simulink model "Position_Control_Sim_01"  (R2025b)
settings: Solver=FixedStepAuto  StartTime=0.0  StopTime=inf  FixedStep=time_step  RelTol=1e-3
values from neighbouring files (symbols this model uses):
  I_max_XY = 5    [Position_Control_Main.m]
  I_max_Z = 1    [Position_Control_Main.m]
  MOT_THST_HOVER_MCS = 1470    [Position_Control_Main.m]
  STABILIZE = 1100    [Position_Control_Main.m]
  time_step = 1/80    (= 0.0125)    [Position_Control_Main.m]
undefined symbols (not defined in the file or in its folder): Data, Data_SL_Info, DiscIntNeverNeededParam
libraries: robotlib x5, sharedtransform x1, aerolibanimutils x1
settings Model: Creator=lirangoshen  LastModifiedBy=lirangoshen
settings DataIOCC: LimitDataPoints=on  MaxDataPoints=10000
settings OptimizationCC: EnhancedBackFolding=on  PassReuseOutputArgsAs=Individual arguments  ZeroExternalMemoryAtStartup=off  ZeroInternalMemoryAtStartup=off  MaxStackSize=64  OptimizeBlockOrder=speed  DifferentSizesBufferReuse=on  OptimizationCustomize=off  EfficientTunableParamExpr=on
settings DebuggingCC: ParameterTunabilityLossMsg=error
settings HardwareCC: ProdBitPerPointer=32.0  ProdBitPerSizeT=32.0  ProdBitPerPtrDiffT=32.0  ProdLargestAtomicFloat=None  ProdIntDivRoundTo=Undefined  ProdEndianess=Unspecified  ProdWordSize=32.0  ProdHWDeviceType=Generic->Unspecified (assume 32-bit Generic)
settings SFSimCC: MATLABDynamicMemAlloc=off
settings RTWCC: SystemTargetFile=ert.tlc  HardwareBoard=Robot Operating System (ROS)  TLCOptions="-aInlineSetEventsForThisBaseRateFcn=TLC_FALSE -aSuppressMultiTaskScheduler=TLC_FALSE  -aRateBasedStepFcn=0"  TemplateMakefile=ert_default_tmf  Toolchain=Catkin  TargetLang=C++  GPUComputeCapability=3.5  Description=Embedded Coder
settings CodeAppCC: ForceParamTrailComments=on  IgnoreCustomStorageClasses=off  OperatorAnnotations=on  SimulinkDataObjDesc=on  SFDataObjDesc=on  InsertBlockDesc=on
settings ERTTargetCC: InlinedParameterPlacement=Hierarchical  DynamicArrayContainerType=coder::array

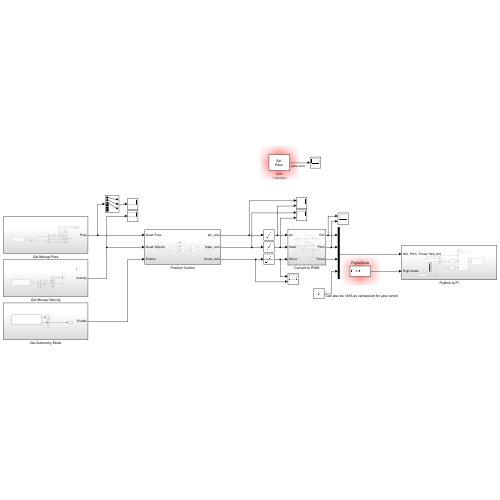
[thumbnail: Simulink's stored preview of the top-level diagram]
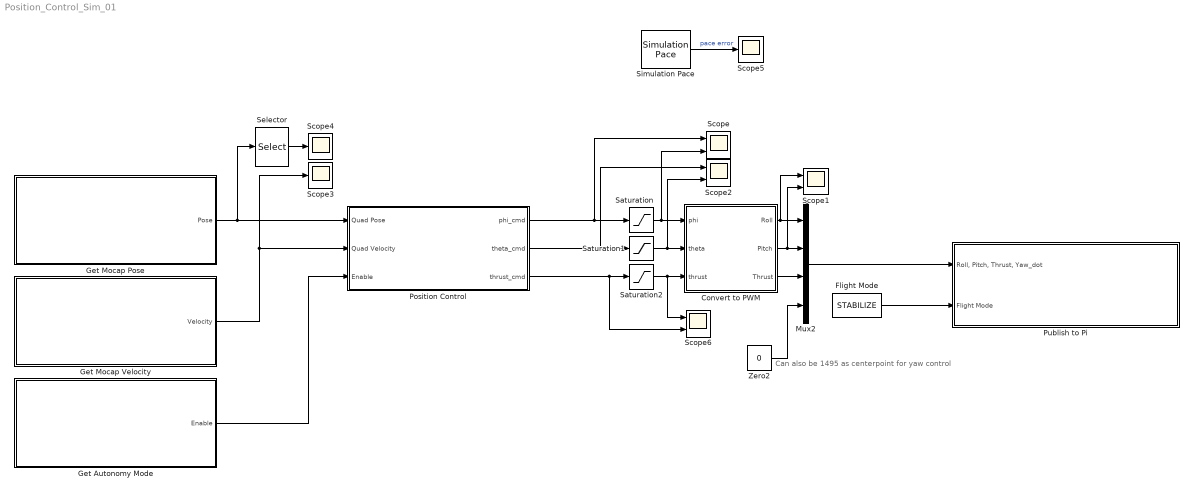
== system Position_Control_Sim_01 ==
  note: Can also be 1495 as centerpoint for yaw control
  Convert to PWM : Subsystem
  Flight Mode : Constant  Value=STABILIZE  OutDataTypeStr=Inherit: Inherit via back propagation
  Get Autonomy Mode : Subsystem
  Get Mocap Pose : Subsystem
  Get Mocap Velocity : Subsystem
  Mux2 : Mux
  Position Control : Subsystem
  Publish to Pi : Subsystem
  Saturation : Saturate  UpperLimit=10  LowerLimit=-10
  Saturation1 : Saturate  UpperLimit=10  LowerLimit=-10
  Saturation2 : Saturate  UpperLimit=3  LowerLimit=-3
  Scope{,1..2,6} (4 alike) : Scope  NumInputPorts=2
      Scope settings: ActiveDisplayYMinimum=-38.87191  ActiveDisplayYMaximum=29.85251
      Scope1 settings: ActiveDisplayYMinimum=1289.66667  ActiveDisplayYMaximum=1706.33333  DataLoggingVariableName=ScopeData2
      Scope2 settings: ActiveDisplayYMinimum=-6.82058  ActiveDisplayYMaximum=8.21599  DataLoggingVariableName=ScopeData3
      Scope6 settings: ActiveDisplayYMinimum=-6.19589  ActiveDisplayYMaximum=6.86106  DataLoggingVariableName=ScopeData7
  Scope3 : Scope
      settings: ActiveDisplayYMinimum=-0.74653  ActiveDisplayYMaximum=0.88268  DataLoggingVariableName=ScopeData4
  Scope4 : Scope
      settings: ActiveDisplayYMinimum=-0.65562  ActiveDisplayYMaximum=1.49202  DataLoggingVariableName=ScopeData5
  Scope5 : Scope
      settings: ActiveDisplayYMinimum=-1  ActiveDisplayYMaximum=1  DataLoggingVariableName=ScopeData6
  Selector : Selector  InputPortWidth=6  IndexOptions=Index vector (dialog)  Indices=1:3  OutputSizes=1
  Simulation Pace : aerolibanimutils/Simulation Pace  SimulationPace=1  SleepMode=Auto  OutputPaceError=on  SampleTime=time_step
  Zero2 : Constant  Value=0  OutDataTypeStr=Inherit: Inherit via back propagation
  wires:
  Flight Mode/1 -> Publish to Pi/2(Flight Mode)
  Position Control/3(thrust_cmd) -> Scope6/2, Saturation2/1
  Convert to PWM/3(Thrust) -> Mux2/3
  Saturation/1 -> Scope/2, Convert to PWM/1(phi)
  Get Mocap Pose/1(Pose) -> Selector/1, Position Control/1(Quad Pose)
  Get Mocap Velocity/1(Velocity) -> Position Control/2(Quad Velocity), Scope3/1
  Convert to PWM/2(Pitch) -> Scope1/2, Mux2/2
  Saturation1/1 -> Scope2/2, Convert to PWM/2(theta)
  Position Control/2(theta_cmd) -> Scope2/1, Saturation1/1
  Saturation2/1 -> Scope6/1, Convert to PWM/3(thrust)
  Zero2/1 -> Mux2/4
  Mux2/1 -> Publish to Pi/1("Roll, Pitch, Thrust, Yaw_dot")
  Selector/1 -> Scope4/1
  Simulation Pace/1 -> Scope5/1  "pace error"
  Get Autonomy Mode/1(Enable) -> Position Control/3(Enable)
  Convert to PWM/1(Roll) -> Mux2/1, Scope1/1
  Position Control/1(phi_cmd) -> Scope/1, Saturation/1

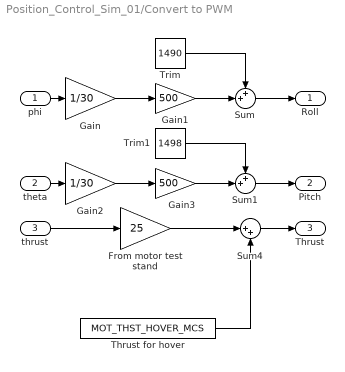
== system Position_Control_Sim_01/Convert to PWM ==
  phi : Inport
  theta : Inport  Port=2
  thrust : Inport  Port=3
  From motor test stand : Gain  Gain=25
  Gain : Gain  Gain=1/30
  Gain1 : Gain  Gain=500
  Gain2 : Gain  Gain=1/30
  Gain3 : Gain  Gain=500
  Sum : Sum  Inputs=++|
  Sum1 : Sum  Inputs=++|
  Sum4 : Sum  Inputs=|++
  Thrust for hover : Constant  Value=MOT_THST_HOVER_MCS
  Trim : Constant  Value=1490
  Trim1 : Constant  Value=1498
  Roll : Outport
  Pitch : Outport  Port=2
  Thrust : Outport  Port=3
  wires:
  phi/1 -> Gain/1
  Gain/1 -> Gain1/1
  Gain1/1 -> Sum/2
  theta/1 -> Gain2/1
  Gain2/1 -> Gain3/1
  Gain3/1 -> Sum1/2
  Sum1/1 -> Pitch/1
  Sum/1 -> Roll/1
  Trim/1 -> Sum/1
  Sum4/1 -> Thrust/1
  Thrust for hover/1 -> Sum4/2
  From motor test stand/1 -> Sum4/1
  Trim1/1 -> Sum1/1
  thrust/1 -> From motor test stand/1

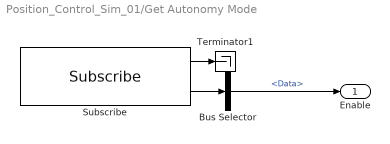
== system Position_Control_Sim_01/Get Autonomy Mode ==
  Bus Selector : BusSelector  OutputSignals=Data
  Subscribe : robotlib/Subscribe  topicSource=Select from ROS network  topic=/autonomy_enable  messageType=std_msgs/Bool  SampleTime=-1  legacyBusStruct=off  messageQueueLength=1
  Terminator1 : Terminator
  Enable : Outport
  wires:
  Subscribe/1 -> Terminator1/1
  Subscribe/2 -> Bus Selector/1
  Bus Selector/1 -> Enable/1  "<Data>"

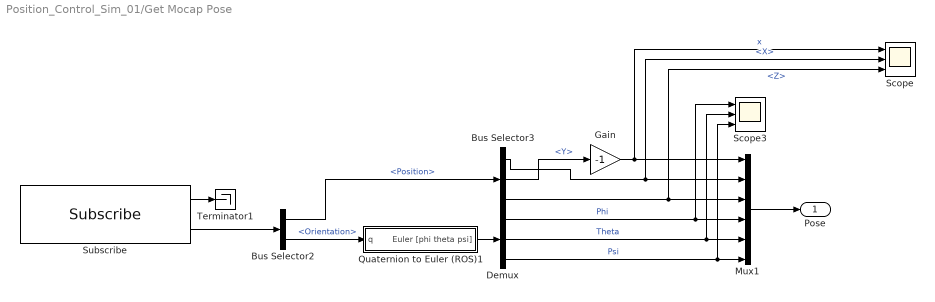
== system Position_Control_Sim_01/Get Mocap Pose ==
  Bus Selector2 : BusSelector  OutputSignals=Pose.Position,Pose.Orientation
  Bus Selector3 : BusSelector  OutputSignals=X,Y,Z
  Demux : Demux  Outputs=3
  Gain : Gain  Gain=-1
  Mux1 : Mux  Inputs=6
  Quaternion to Euler (ROS)1 : Subsystem
  Scope : Scope  NumInputPorts=3
      settings: ActiveDisplayYMinimum=-2.27566  ActiveDisplayYMaximum=3.58367
  Scope3 : Scope  NumInputPorts=3
      settings: ActiveDisplayYMinimum=-0.14354  ActiveDisplayYMaximum=0.09854
  Subscribe : robotlib/Subscribe  topicSource=Select from ROS network  topic=/vrpn_client_node/Quad1/pose  messageType=geometry_msgs/PoseStamped  SampleTime=-1  legacyBusStruct=off  messageQueueLength=1
  Terminator1 : Terminator
  Pose : Outport
  wires:
  Demux/3 -> Scope3/3, Mux1/6  "Psi"
  Demux/2 -> Scope3/2, Mux1/5  "Theta"
  Bus Selector3/1 -> Scope/2, Mux1/2  "<X>"
  Bus Selector3/3 -> Scope/3, Mux1/3  "<Z>"
  Bus Selector2/1 -> Bus Selector3/1  "<Position>"
  Subscribe/2 -> Bus Selector2/1
  Bus Selector2/2 -> Quaternion to Euler (ROS)1/1(q)  "<Orientation>"
  Demux/1 -> Scope3/1, Mux1/4  "Phi"
  Bus Selector3/2 -> Gain/1  "<Y>"
  Quaternion to Euler (ROS)1/1(Euler [phi theta psi]) -> Demux/1
  Subscribe/1 -> Terminator1/1
  Mux1/1 -> Pose/1
  Gain/1 -> Scope/1, Mux1/1  "x"

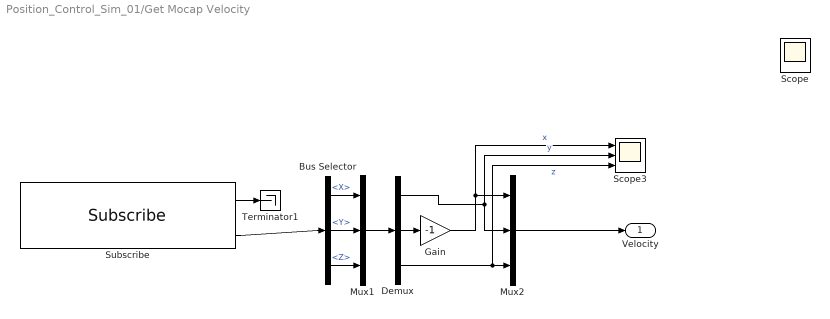
== system Position_Control_Sim_01/Get Mocap Velocity ==
  Bus Selector : BusSelector  OutputSignals=Twist.Linear.X,Twist.Linear.Y,Twist.Linear.Z
  Demux : Demux  Outputs=3
  Gain : Gain  Gain=-1
  Mux1 : Mux  Inputs=3
  Mux2 : Mux  Inputs=3
  Scope : Scope  NumInputPorts=3
      settings: ActiveDisplayYMinimum=-2.34583  ActiveDisplayYMaximum=1.6717
  Scope3 : Scope  NumInputPorts=3
      settings: ActiveDisplayYMinimum=-2.23805  ActiveDisplayYMaximum=2.22342
  Subscribe : robotlib/Subscribe  topicSource=Select from ROS network  topic=/vrpn_velocity/optitrack_frame/filtered  messageType=geometry_msgs/TwistStamped  SampleTime=-1  legacyBusStruct=off  messageQueueLength=1
  Terminator1 : Terminator
  Velocity : Outport
  wires:
  Subscribe/1 -> Terminator1/1
  Subscribe/2 -> Bus Selector/1
  Bus Selector/1 -> Mux1/1  "<X>"
  Bus Selector/2 -> Mux1/2  "<Y>"
  Bus Selector/3 -> Mux1/3  "<Z>"
  Mux1/1 -> Demux/1
  Demux/2 -> Gain/1
  Demux/1 -> Mux2/2, Scope3/2  "y"
  Gain/1 -> Scope3/1, Mux2/1  "x"
  Demux/3 -> Scope3/3, Mux2/3  "z"
  Mux2/1 -> Velocity/1

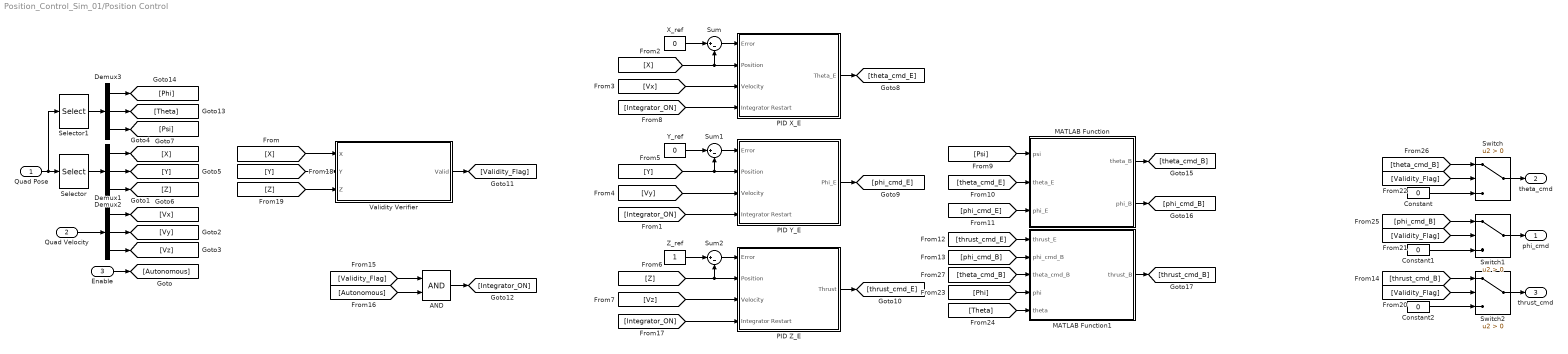
== system Position_Control_Sim_01/Position Control ==
  Quad Pose : Inport
  Quad Velocity : Inport  Port=2
  Enable : Inport  Port=3
  AND : Logic  IconShape=distinctive  AllPortsSameDT=off  OutDataTypeStr=boolean
  Constant : Constant  Value=0
  Constant1 : Constant  Value=0
  Constant2 : Constant  Value=0
  Demux1 : Demux  Outputs=3
  Demux2 : Demux  Outputs=3
  Demux3 : Demux  Outputs=3
  MATLAB Function : MATLAB Function  TreatAsAtomicUnit=on
  MATLAB Function1 : MATLAB Function  TreatAsAtomicUnit=on
  PID X_E : Subsystem
  PID Y_E : Subsystem
  PID Z_E : Subsystem
  Selector : Selector  InputPortWidth=6  IndexOptions=Index vector (dialog)  Indices=[1 2 3]  OutputSizes=1
  Selector1 : Selector  InputPortWidth=6  IndexOptions=Index vector (dialog)  Indices=[4 5 6]  OutputSizes=1
  Sum : Sum  Inputs=|+-
  Sum1 : Sum  Inputs=|+-
  Sum2 : Sum  Inputs=|+-
  Switch : Switch  Criteria=u2 > Threshold  SaturateOnIntegerOverflow=off  InputSameDT=off
  Switch1 : Switch  Criteria=u2 > Threshold  SaturateOnIntegerOverflow=off  InputSameDT=off
  Switch2 : Switch  Criteria=u2 > Threshold  SaturateOnIntegerOverflow=off  InputSameDT=off
  Validity Verifier : Subsystem
  X_ref : Constant  Value=0
  Y_ref : Constant  Value=0
  Z_ref : Constant
  phi_cmd : Outport
  theta_cmd : Outport  Port=2
  thrust_cmd : Outport  Port=3
  wires:
  Quad Pose/1 -> Selector1/1, Selector/1
  Selector/1 -> Demux2/1
  X_ref/1 -> Sum/1
  Y_ref/1 -> Sum1/1
  PID Z_E/1(Thrust) -> [thrust_cmd_E]
  Sum/1 -> PID X_E/1(Error)
  [Vx] -> PID X_E/3(Velocity)
  Sum1/1 -> PID Y_E/1(Error)
  [Vy] -> PID Y_E/3(Velocity)
  Enable/1 -> [Autonomous]
  [Integrator_ON] -> PID Y_E/4(Integrator Restart)
  [Integrator_ON] -> PID X_E/4(Integrator Restart)
  Quad Velocity/1 -> Demux1/1
  Demux1/1 -> [Vx]
  Demux1/2 -> [Vy]
  Demux1/3 -> [Vz]
  Demux2/1 -> [X]
  Demux2/2 -> [Y]
  Demux2/3 -> [Z]
  [X] -> PID X_E/2(Position), Sum/2
  [Y] -> PID Y_E/2(Position), Sum1/2
  Z_ref/1 -> Sum2/1
  Sum2/1 -> PID Z_E/1(Error)
  [Z] -> Sum2/2, PID Z_E/2(Position)
  [Vz] -> PID Z_E/3(Velocity)
  [Integrator_ON] -> PID Z_E/4(Integrator Restart)
  Selector1/1 -> Demux3/1
  [Psi] -> MATLAB Function/1(psi)
  PID X_E/1(Theta_E) -> [theta_cmd_E]
  PID Y_E/1(Phi_E) -> [phi_cmd_E]
  Switch/1 -> theta_cmd/1
  MATLAB Function/1(theta_B) -> [theta_cmd_B]
  [theta_cmd_E] -> MATLAB Function/2(theta_E)
  [phi_cmd_E] -> MATLAB Function/3(phi_E)
  Switch1/1 -> phi_cmd/1
  [thrust_cmd_E] -> MATLAB Function1/1(thrust_E)
  [theta_cmd_B] -> MATLAB Function1/3(theta_cmd_B)
  Validity Verifier/1(Valid) -> [Validity_Flag]
  [Validity_Flag] -> AND/1
  [Autonomous] -> AND/2
  AND/1 -> [Integrator_ON]
  MATLAB Function1/1(thrust_B) -> [thrust_cmd_B]
  Switch2/1 -> thrust_cmd/1
  [Validity_Flag] -> Switch2/2
  [Validity_Flag] -> Switch1/2
  MATLAB Function/2(phi_B) -> [phi_cmd_B]
  [Validity_Flag] -> Switch/2
  Demux3/2 -> [Theta]
  Demux3/3 -> [Psi]
  Demux3/1 -> [Phi]
  [Phi] -> MATLAB Function1/4(phi)
  [Theta] -> MATLAB Function1/5(theta)
  [phi_cmd_B] -> MATLAB Function1/2(phi_cmd_B)
  [phi_cmd_B] -> Switch1/1
  Constant/1 -> Switch/3
  Constant1/1 -> Switch1/3
  [theta_cmd_B] -> Switch/1
  [thrust_cmd_B] -> Switch2/1
  Constant2/1 -> Switch2/3
  [Y] -> Validity Verifier/2(Y)
  [X] -> Validity Verifier/1(X)
  [Z] -> Validity Verifier/3(Z)

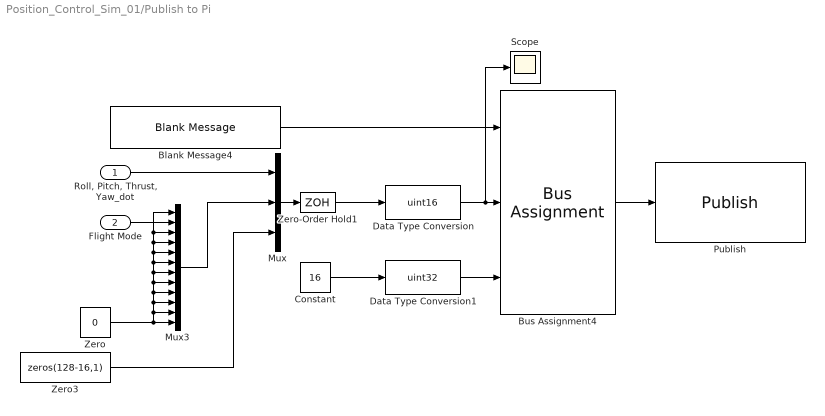
== system Position_Control_Sim_01/Publish to Pi ==
  "Roll, Pitch, Thrust, Yaw_dot" : Inport
  Flight Mode : Inport  Port=2
  Blank Message4 : robotlib/Blank Message  messageClass=Message  entityType=std_msgs/UInt16MultiArray  messageType=std_msgs/UInt16MultiArray  SampleTime=-1  legacyBusStruct=off
  Bus Assignment4 : BusAssignment  AssignedSignals=Data,Data_SL_Info.CurrentLength
  Constant : Constant  Value=16
  Data Type Conversion : DataTypeConversion  OutDataTypeStr=uint16  SaturateOnIntegerOverflow=off  RndMeth=Floor
  Data Type Conversion1 : DataTypeConversion  OutDataTypeStr=uint32  SaturateOnIntegerOverflow=off  RndMeth=Floor
  Mux : Mux  Inputs=3
  Mux3 : Mux  Inputs=12
  Publish : robotlib/Publish  topicSource=Specify your own  topic=quad_commands  messageType=std_msgs/UInt16MultiArray  legacyBusStruct=off  messageQueueLength=1
  Scope : Scope
      settings: ActiveDisplayYMinimum=-208  ActiveDisplayYMaximum=1872  DataLoggingVariableName=ScopeData5
  Zero : Constant  Value=0  OutDataTypeStr=Inherit: Inherit via back propagation
  Zero-Order Hold1 : ZeroOrderHold  SampleTime=-1
  Zero3 : Constant  Value=zeros(128-16,1)  OutDataTypeStr=Inherit: Inherit via back propagation
  wires:
  Data Type Conversion1/1 -> Bus Assignment4/3
  Zero/1 -> Mux3/1, Mux3/3, Mux3/4, Mux3/5, Mux3/6, Mux3/7, Mux3/8, Mux3/9, Mux3/10, Mux3/11, Mux3/12
  Mux3/1 -> Mux/2
  Mux/1 -> Zero-Order Hold1/1
  Bus Assignment4/1 -> Publish/1
  Blank Message4/1 -> Bus Assignment4/1
  Zero-Order Hold1/1 -> Data Type Conversion/1
  Zero3/1 -> Mux/3
  Constant/1 -> Data Type Conversion1/1
  "Roll, Pitch, Thrust, Yaw_dot"/1 -> Mux/1
  Data Type Conversion/1 -> Scope/1, Bus Assignment4/2
  Flight Mode/1 -> Mux3/2

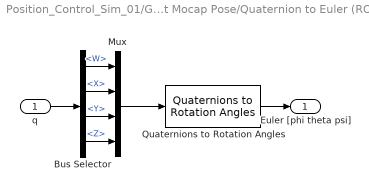
== system Position_Control_Sim_01/Get Mocap Pose/Quaternion to Euler (ROS)1 ==
  q : Inport
  Bus Selector : BusSelector  OutputSignals=W,X,Y,Z
  Mux : Mux
  Quaternions to Rotation Angles : sharedtransform/Quaternions to Rotation Angles  rotationOrder=XYZ  aMode=aMode
  Euler [phi theta psi] : Outport
  wires:
  Mux/1 -> Quaternions to Rotation Angles/1
  q/1 -> Bus Selector/1
  Bus Selector/1 -> Mux/1  "<W>"
  Bus Selector/2 -> Mux/2  "<X>"
  Bus Selector/3 -> Mux/3  "<Y>"
  Bus Selector/4 -> Mux/4  "<Z>"
  Quaternions to Rotation Angles/1 -> Euler [phi theta psi]/1

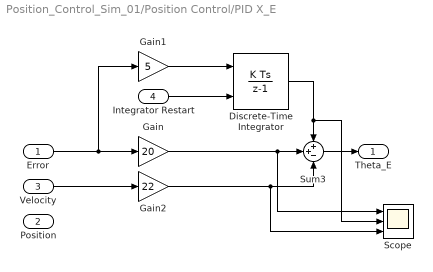
== system Position_Control_Sim_01/Position Control/PID X_E ==
  Error : Inport
  Position : Inport  Port=2
  Velocity : Inport  Port=3
  Integrator Restart : Inport  Port=4
  Discrete-Time Integrator : DiscreteIntegrator  ExternalReset=rising  SampleTime=-1  LimitOutput=on  UpperSaturationLimit=I_max_XY  LowerSaturationLimit=-I_max_XY  ICPrevOutput=DiscIntNeverNeededParam  ICPrevScaledInput=DiscIntNeverNeededParam
  Gain : Gain  Gain=20
  Gain1 : Gain  Gain=5
  Gain2 : Gain  Gain=22
  Scope : Scope  NumInputPorts=3
      settings: ActiveDisplayYMinimum=-13.86541  ActiveDisplayYMaximum=8.81324  DataLoggingVariableName=ScopeData2
  Sum3 : Sum  Inputs=++-
  Theta_E : Outport
  wires:
  Error/1 -> Gain1/1, Gain/1
  Sum3/1 -> Theta_E/1
  Discrete-Time Integrator/1 -> Scope/2, Sum3/1
  Gain2/1 -> Scope/3, Sum3/3
  Gain/1 -> Scope/1, Sum3/2
  Integrator Restart/1 -> Discrete-Time Integrator/2
  Velocity/1 -> Gain2/1
  Gain1/1 -> Discrete-Time Integrator/1

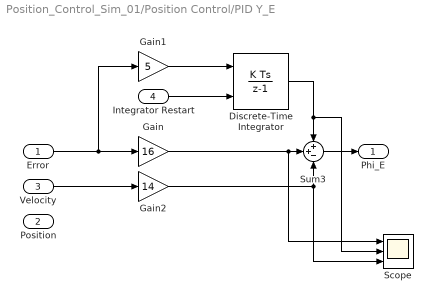
== system Position_Control_Sim_01/Position Control/PID Y_E ==
  Error : Inport
  Position : Inport  Port=2
  Velocity : Inport  Port=3
  Integrator Restart : Inport  Port=4
  Discrete-Time Integrator : DiscreteIntegrator  ExternalReset=rising  SampleTime=-1  LimitOutput=on  UpperSaturationLimit=I_max_XY  LowerSaturationLimit=-I_max_XY  ICPrevOutput=DiscIntNeverNeededParam  ICPrevScaledInput=DiscIntNeverNeededParam
  Gain : Gain  Gain=16
  Gain1 : Gain  Gain=5
  Gain2 : Gain  Gain=14
  Scope : Scope  NumInputPorts=3
      settings: ActiveDisplayYMinimum=-36.68782  ActiveDisplayYMaximum=41.34119
  Sum3 : Sum  Inputs=++-
  Phi_E : Outport
  wires:
  Error/1 -> Gain1/1, Gain/1
  Sum3/1 -> Phi_E/1
  Discrete-Time Integrator/1 -> Scope/2, Sum3/1
  Gain2/1 -> Sum3/3, Scope/3
  Gain/1 -> Scope/1, Sum3/2
  Integrator Restart/1 -> Discrete-Time Integrator/2
  Velocity/1 -> Gain2/1
  Gain1/1 -> Discrete-Time Integrator/1

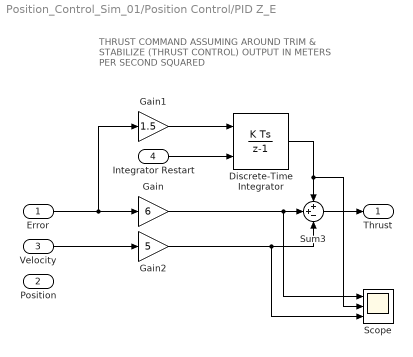
== system Position_Control_Sim_01/Position Control/PID Z_E ==
  note: THRUST COMMAND ASSUMING AROUND TRIM
      | & STABILIZE (THRUST CONTROL)
      |
      | OUTPUT IN METERS PER SECOND SQUARED
  Error : Inport
  Position : Inport  Port=2
  Velocity : Inport  Port=3
  Integrator Restart : Inport  Port=4
  Discrete-Time Integrator : DiscreteIntegrator  ExternalReset=rising  SampleTime=-1  LimitOutput=on  UpperSaturationLimit=I_max_Z  LowerSaturationLimit=-I_max_Z  ICPrevOutput=DiscIntNeverNeededParam  ICPrevScaledInput=DiscIntNeverNeededParam
  Gain : Gain  Gain=6
  Gain1 : Gain  Gain=1.5
  Gain2 : Gain  Gain=5
  Scope : Scope  NumInputPorts=3
      settings: ActiveDisplayYMinimum=-6.37854  ActiveDisplayYMaximum=7.05147  DataLoggingVariableName=ScopeData3
  Sum3 : Sum  Inputs=++-
  Thrust : Outport
  wires:
  Velocity/1 -> Gain2/1
  Error/1 -> Gain1/1, Gain/1
  Gain/1 -> Scope/1, Sum3/2
  Sum3/1 -> Thrust/1
  Gain1/1 -> Discrete-Time Integrator/1
  Gain2/1 -> Scope/3, Sum3/3
  Discrete-Time Integrator/1 -> Scope/2, Sum3/1
  Integrator Restart/1 -> Discrete-Time Integrator/2

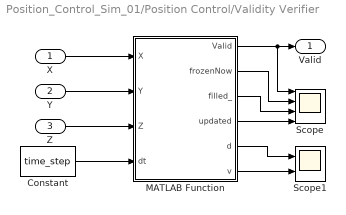
== system Position_Control_Sim_01/Position Control/Validity Verifier ==
  X : Inport
  Y : Inport  Port=2
  Z : Inport  Port=3
  Constant : Constant  Value=time_step
  MATLAB Function : MATLAB Function  TreatAsAtomicUnit=on
  Scope : Scope  NumInputPorts=4
      settings: ActiveDisplayYMinimum=-1.375  ActiveDisplayYMaximum=12.375
  Scope1 : Scope  NumInputPorts=2
      settings: ActiveDisplayYMinimum=-9.28189  ActiveDisplayYMaximum=73.53703  DataLoggingVariableName=ScopeData2
  Valid : Outport
  wires:
  X/1 -> MATLAB Function/1(X)
  Y/1 -> MATLAB Function/2(Y)
  Z/1 -> MATLAB Function/3(Z)
  Constant/1 -> MATLAB Function/4(dt)
  MATLAB Function/1(Valid) -> Scope/1, Valid/1
  MATLAB Function/2(frozenNow) -> Scope/2
  MATLAB Function/3(filled_) -> Scope/3
  MATLAB Function/4(updated) -> Scope/4
  MATLAB Function/5(d) -> Scope1/1
  MATLAB Function/6(v) -> Scope1/2

== matlab function Position_Control_Sim_01/Position Control/MATLAB Function1 ==
  data: thrust_E input; thrust_B output; phi_cmd_B input; theta_cmd_B input; phi input; theta input
function thrust_B  = Correct_for_tilt(thrust_E, phi_cmd_B, theta_cmd_B, phi, theta)

alpha = 0.5;

phi_ff = alpha*phi+(1-alpha)*phi_cmd_B;
theta_ff = alpha*theta+(1-alpha)*theta_cmd_B;

thrust_B = thrust_E/cosd(theta_ff)/cosd(phi_ff);

== matlab function Position_Control_Sim_01/Position Control/MATLAB Function ==
  data: psi input; theta_B output; theta_E input; phi_E input; phi_B output
function [theta_B, phi_B] = Rotate_by_yaw(psi, theta_E, phi_E)

theta_B = - phi_E*sin(psi) - theta_E*cos(psi);
phi_B   = - phi_E*cos(psi) + theta_E*sin(psi);

== matlab function Position_Control_Sim_01/Position Control/Validity Verifier/MATLAB Function ==
  data: X input; Valid output; Y input; Z input; dt input; frozenNow output; filled_ output; updated output; d output; v output
function [Valid, frozenNow, filled_, updated, d, v]  = fcn(X, Y, Z, dt)

% Validity checker for mocap pose
% Invalid if:
%  - speed > 10 m/s between samples
%  - position unchanged for N timesteps
% Recovery:
%  - after updates resume, require M consecutive good updates before Valid=1

% ---- Tunables ----
VMAX = 20.0;      % m/s
N    = 10;         % frozen threshold (timesteps)
M    = 5;         % recovery required good updates

K = max(N,M)+1;            % max(N,M) = 5 for your initial values

% ---- Persistent state ----
persistent bufX bufY bufZ idx filled inLost goodCnt

if isempty(bufX)
    bufX    = zeros(1, K);
    bufY    = zeros(1, K);
    bufZ    = zeros(1, K);
    idx     = uint8(1);
    filled  = uint8(0);
    inLost  = false;
    goodCnt = uint8(0);
end

% If first sample, initialize history and return valid
if filled == 0
    bufX(idx) = X; bufY(idx) = Y; bufZ(idx) = Z;
    filled = uint8(1);
    idx = uint8(2);
    Valid = true;
    frozenNow = false;
    filled_ = uint8(0);
    updated = false;
    d = -1;
    v = -1;
    return;
end

% Previous sample index
prevIdx = idx - 1;
if prevIdx == 0
    prevIdx = uint8(K);
end

% Compute delta and implied speed from previous sample
dx = X - bufX(prevIdx);
dy = Y - bufY(prevIdx);
dz = Z - bufZ(prevIdx);
d  = sqrt(dx*dx + dy*dy + dz*dz);

v = d / dt;
updated = (d > 1e-6);

% ---- Frozen detection using last (N+1) samples ----
frozenNow = false;
if filled >= uint8(N+1)
    % Check if current sample is (approximately) equal to each of last N samples
    % i.e., no meaningful movement for N consecutive intervals
    frozenNow = true;
    j = prevIdx;
    for k = 1:N
        ddx = X - bufX(j);
        ddy = Y - bufY(j);
        ddz = Z - bufZ(j);
        if sqrt(ddx*ddx + ddy*ddy + ddz*ddz) > 1e-6
            frozenNow = false;
            break;
        end
        j = j - 1;
        if j == 0
            j = uint8(K);
        end
    end
end

% ---- Validity / recovery logic ----
if ~inLost
    if (v > VMAX) || frozenNow
        inLost  = true;
        goodCnt = uint8(0);
        Valid   = false;
    else
        Valid = true;
    end
else
    % Lost: require M consecutive "good updates" to re-trust
    if updated && (v <= VMAX)
        if goodCnt < uint8(255)
            goodCnt = goodCnt + 1;
        end
        if goodCnt >= uint8(M)
            inLost  = false;
            goodCnt = uint8(0);
            Valid   = true;
        else
            Valid = false;
        end
    else
        % Still bad or still frozen; reset recovery counter on outlier
        if v > VMAX
            goodCnt = uint8(0);
        end
        Valid = false;
    end
end

% ---- Push current sample into ring buffer ----
bufX(idx) = X; bufY(idx) = Y; bufZ(idx) = Z;

if filled < uint8(K)
    filled = filled + 1;
end

idx = idx + 1;
if idx > uint8(K)
    idx = uint8(1);
end

filled_ = filled;
end
